simulink model "equalize_the_step_responses"  (R2022b)
settings: Solver=FixedStepAuto  StartTime=0.0  StopTime=2  FixedStep=0.002  RelTol=1e-3
libraries: simulink x2
settings Model: Creator=mrxmi  LastModifiedBy=mrxmi

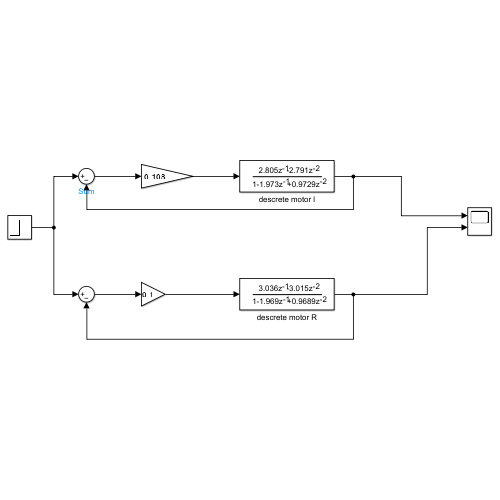
[thumbnail: Simulink's stored preview of the top-level diagram]
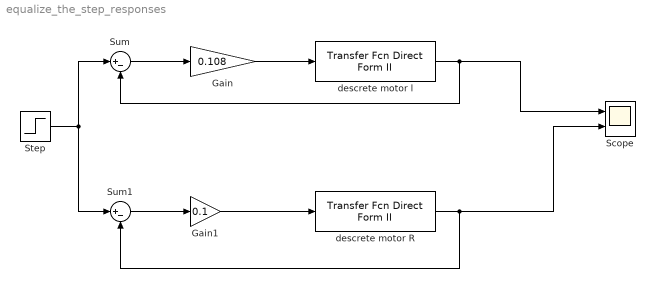
== system equalize_the_step_responses ==
  Gain : Gain  Gain=0.108
  Gain1 : Gain  Gain=0.1
  Scope : Scope  NumInputPorts=2
  Step : Step  After=400  SampleTime=0
  Sum : Sum  Inputs=|+-
  Sum1 : Sum  Inputs=|+-
  descrete motor R : simulink/Additional Math & Discrete/Additional Discrete/Transfer Fcn Direct Form II  NumCoefVec=[0 3.036 -3.015]  DenCoefVec=[-1.969 0.9689]  vinit=0.0  DoSatur=off
  descrete motor l : simulink/Additional Math & Discrete/Additional Discrete/Transfer Fcn Direct Form II  NumCoefVec=[0 2.805 -2.791]  DenCoefVec=[-1.973 0.9729]  vinit=0.0  DoSatur=off
  wires:
  Step/1 -> Sum/1, Sum1/1
  Sum/1 -> Gain/1
  Gain/1 -> descrete motor l/1
  descrete motor l/1 -> Scope/1, Sum/2
  descrete motor R/1 -> Scope/2, Sum1/2
  Sum1/1 -> Gain1/1
  Gain1/1 -> descrete motor R/1
